simulink subsystem "Twist_Publisher"  (R2022b)
settings: Solver=VariableStepAuto  StartTime=0.0  StopTime=10.0  RelTol=1e-3
undefined symbols (not defined in the file or in its folder): header, twist
libraries: ros2lib x2
settings Model: Creator=hayden  LastModifiedBy=hollis
settings ModelReferenceCC: EnableRefExpFcnMdlSchedulingChecks=on

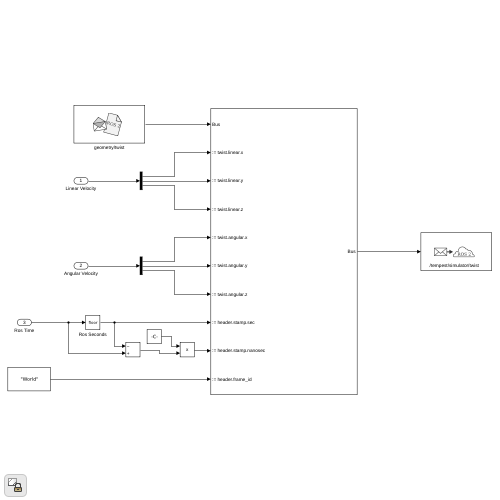
[thumbnail: Simulink's stored preview of the top-level diagram]
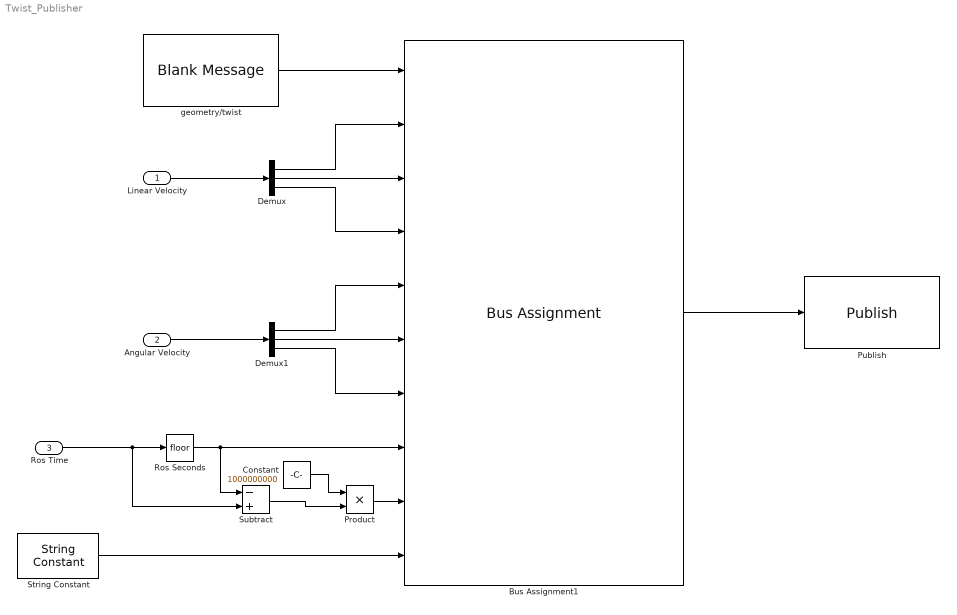
== system Twist_Publisher ==
  Linear Velocity : Inport
  Angular Velocity : Inport  Port=2
  Ros Time : Inport  Port=3
  Bus Assignment1 : BusAssignment  AssignedSignals=twist.linear.x,twist.linear.y,twist.linear.z,twist.angular.x,twist.angular.y,twist.angular.z,header.stamp.sec,header.stamp.nanosec,header.frame_id
  Constant : Constant  Value=1000000000
  Demux : Demux  Outputs=3
  Demux1 : Demux  Outputs=3
  Product : Product
  Publish : ros2lib/Publish  topicSource=Specify your own  topic=/tempest/simulator/twist  messageType=geometry_msgs/Twist  QOSHistory=Keep last  QOSDepth=1  QOSReliability=Reliable  QOSDurability=Volatile
  Ros Seconds : Rounding
  String Constant : StringConstant  String="\"World\""
  Subtract : Sum  Inputs=-+
  geometry/twist : ros2lib/Blank Message  messageClass=Message  entityType=geometry_msgs/TwistStamped  messageType=geometry_msgs/TwistStamped  SampleTime=inf
  wires:
  geometry/twist/1 -> Bus Assignment1/1
  Bus Assignment1/1 -> Publish/1
  Demux/2 -> Bus Assignment1/3
  Demux/1 -> Bus Assignment1/2
  Demux/3 -> Bus Assignment1/4
  Demux1/2 -> Bus Assignment1/6
  Demux1/1 -> Bus Assignment1/5
  Demux1/3 -> Bus Assignment1/7
  Linear Velocity/1 -> Demux/1
  Angular Velocity/1 -> Demux1/1
  Ros Seconds/1 -> Subtract/1, Bus Assignment1/8
  String Constant/1 -> Bus Assignment1/10
  Constant/1 -> Product/1
  Subtract/1 -> Product/2
  Ros Time/1 -> Ros Seconds/1, Subtract/2
  Product/1 -> Bus Assignment1/9
